simulink model "InvertedPendulum_RealSystem_final"  (R2018a)
settings: Solver=FixedStepDiscrete  StartTime=0.0  StopTime=inf  FixedStep=0.005  RelTol=1e-3
values from neighbouring files (symbols this model uses):
  K_realsetup = lqr(system_open,Q_realsetup,R_realsetup)    [InvertedPendulum.m]
  Omega_c = 25*2*pi    (= 157.079632679)    [InvertedPendulum.m]
  reference_State = [1;0;0;0]    [INVERTEDPENDULUM.m]    (also in InvertedPendulum.m = [0;0;0;0])
  T_s = 1/200    (= 0.005)    [InvertedPendulum.m]
  V_max = 5    [InvertedPendulum.m]
undefined symbols (not defined in the file or in its folder): National_Instruments, PCI
libraries: sldrtlib x2, simulink_extras x1
settings Model: SimulationMode=external  ExtModeTrigDuration=200000  Creator=magudelo  LastModifiedBy=DeKon
settings SolverCC: InsertRTBMode=Always
settings DataIOCC: LimitDataPoints=on  SaveFormat=Array
settings OptimizationCC: ExpressionDepthLimit=2147483647
settings DebuggingCC: UnderspecifiedInitializationDetection=Classic  MergeDetectMultiDrivingBlocksExec=none  SolverPrmCheckMsg=warning  FcnCallInpInsideContextMsg=warning  StateNameClashWarn=warning  SFUnexpectedBacktrackingDiag=warning  SFNoUnconditionalDefaultTransitionDiag=warning  SFExecutionAtInitializationDiag=none
settings ModelReferenceCC: PropagateSignalLabelsOutOfModel=off
settings RTWCC: SystemTargetFile=sldrt.tlc  TemplateMakefile=sldrt.tmf  Description=Simulink Desktop Real-Time  RTWCompilerOptimization=on
settings CodeAppCC: MaxIdLength=95  StateflowObjectComments=on
settings TargetCC: TargetPreCompLibLocation=C:\Program Files\MATLAB\R2018a\toolbox\sldrt\lib\win64  GeneratePreprocessorConditionals=Use local settings
settings ConfigComp: CovMetricSettings=dw  CovHtmlReporting=on  CovSaveCumulativeToWorkspaceVar=on  CovSaveSingleToWorkspaceVar=on  CovExternalEMLEnable=off

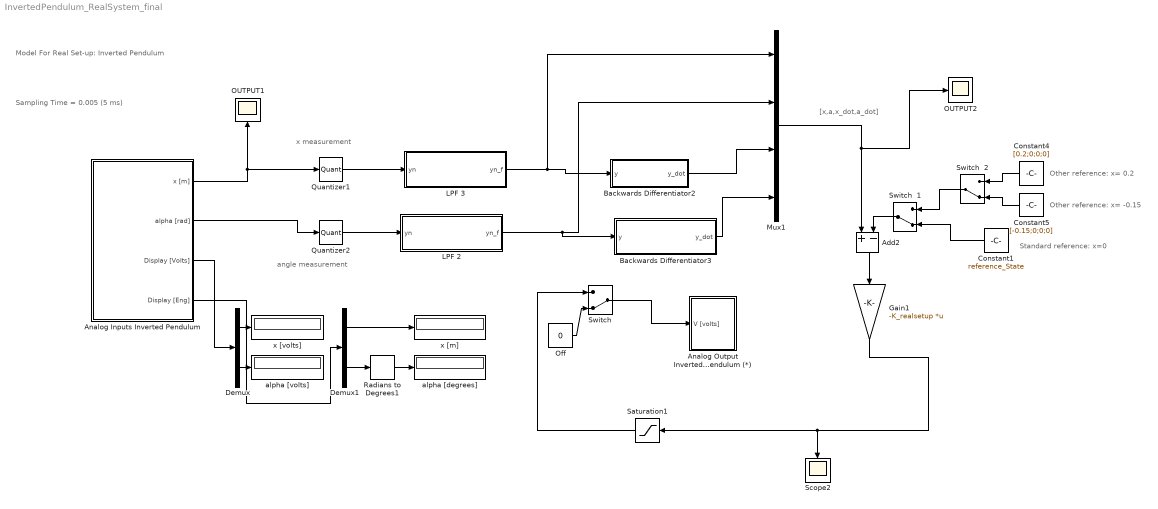
== system InvertedPendulum_RealSystem_final ==
  note: Standard reference: x=0
  note: Other reference: x= 0.2
  note: Model For Real Set-up: Inverted Pendulum
  note: Sampling Time = 0.005 (5 ms)
  note: angle measurement
  note: x measurement
  note: [x,a,x_dot,a_dot]
  note: Other reference: x= -0.15
  Add2 : Sum  Inputs=+-
  Analog Inputs Inverted Pendulum : Subsystem  mask(Analog Inputs. Inverted Pendulum){v2m=0.1033, offset_x=-0.3421, v2r=0.2482, offset_alfa=0.1437}
      mask prompts: v2m "F_x = Convertion factor from Volts to Meters:"; offset_x "Off_x = Offset for the Cart Position [Volts] :"; v2r "F_alpha = Convertion Factor from Volts to Radians :"; offset_alfa "Off_alpha = Offset for the angle of the rob [Volts] :"
      mask help:
      | Remember:
      |    Cart Position (x)           => channel ACH0
      |    Angle of the rod (alpha) => channel ACH1
      |
      |   Cart Position [m] = F_x * ( Cart Position [v] + off_x )
      |   Angle of the rod [rad] = F_alpha * ( Angle of the rod [v] + off_alpha )
  Analog Output Inverted Pendulum (*) : Subsystem  mask(Analog Output - Inverted Pendulum){}
      mask help:
      | Remember
      |    AO 0 => Power Amplifier + Motor
  Backwards Differentiator2 : Subsystem
  Backwards Differentiator3 : Subsystem
  Constant1 : Constant  Value=reference_State
  Constant4 : Constant  Value=[0.2;0;0;0]
  Constant5 : Constant  Value=[-0.15;0;0;0]
  Demux : Demux  Outputs=2
  Demux1 : Demux  Outputs=2
  Gain1 : Gain  Gain=-K_realsetup  Multiplication=Matrix(K*u) (u vector)
  LPF 2 : Subsystem
  LPF 3 : Subsystem
  Mux1 : Mux
  OUTPUT1 : Scope
  OUTPUT2 : Scope
  Off : Constant  Value=0
  Quantizer1 : Quantizer  QuantizationInterval=Q_interval
  Quantizer2 : Quantizer  QuantizationInterval=Q_interval
  Radians to Degrees1 : simulink_extras/Transformations/Radians to Degrees
  Saturation1 : Saturate  UpperLimit=V_max  LowerLimit=-V_max
  Scope2 : Scope
  "Switch  " : ManualSwitch  CurrentSetting=0
  Switch  1 : ManualSwitch  CurrentSetting=0
  Switch  2 : ManualSwitch  CurrentSetting=0
  alpha [degrees] : Display
  alpha [volts] : Display
  x [m] : Display
  x [volts] : Display
  wires:
  Off/1 -> "Switch  "/2
  "Switch  "/1 -> Analog Output Inverted Pendulum (*)/1(V [volts])
  Demux/1 -> x [volts]/1
  Demux1/1 -> x [m]/1
  Demux1/2 -> Radians to Degrees1/1
  Radians to Degrees1/1 -> alpha [degrees]/1
  Analog Inputs Inverted Pendulum/4(Display [Eng]) -> Demux1/1
  Demux/2 -> alpha [volts]/1
  Analog Inputs Inverted Pendulum/3(Display [Volts]) -> Demux/1
  LPF 2/1(yn_f) -> Mux1/2, Backwards Differentiator3/1(y)
  LPF 3/1(yn_f) -> Mux1/1, Backwards Differentiator2/1(y)
  Analog Inputs Inverted Pendulum/2(alpha [rad]) -> Quantizer2/1
  Backwards Differentiator2/1(y_dot) -> Mux1/3
  Analog Inputs Inverted Pendulum/1(x [m]) -> Quantizer1/1, OUTPUT1/1
  Backwards Differentiator3/1(y_dot) -> Mux1/4
  Gain1/1 -> Saturation1/1, Scope2/1
  Mux1/1 -> OUTPUT2/1, Add2/1
  Add2/1 -> Gain1/1
  Saturation1/1 -> "Switch  "/1
  Quantizer1/1 -> LPF 3/1(yn)
  Quantizer2/1 -> LPF 2/1(yn)
  Constant1/1 -> Switch  1/2
  Switch  1/1 -> Add2/2
  Switch  2/1 -> Switch  1/1
  Constant4/1 -> Switch  2/1
  Constant5/1 -> Switch  2/2

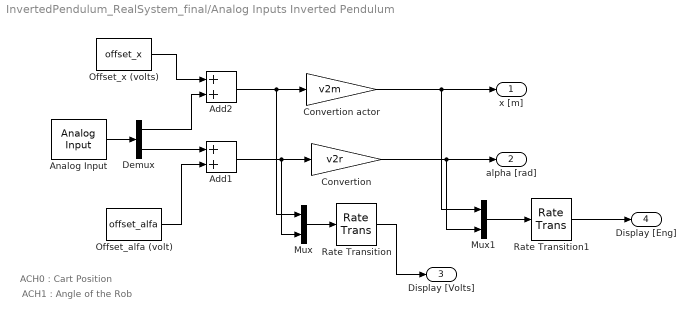
== system InvertedPendulum_RealSystem_final/Analog Inputs Inverted Pendulum ==
  note: ACH0 : Cart Position
  note: ACH1 : Angle of the Rob
  Add1 : Sum
  Add2 : Sum
  Analog Input : sldrtlib/Analog Input  SampleTime=0.005  MaxMissedTicks=10  ShowMissedTicks=off  YieldWhenWaiting=off  DrvName=National_Instruments/PCI-6014  DrvAddress=4294967295  DrvOptions=[1 0 0 0 0 0]  Channels=[1 2]  RangeMode=1  VoltRange=1  DataType=1
      settings: AttributesFormatString=National Instruments\nPCI-6014 [auto]  SourceProductName=Simulink Desktop Real-Time
  "Convertion " : Gain  Gain=v2r
  Convertion actor : Gain  Gain=v2m
  Demux : Demux  Outputs=2
  Mux : Mux  Inputs=2
  Mux1 : Mux  Inputs=2
  Offset_alfa (volt) : Constant  Value=offset_alfa
  Offset_x (volts) : Constant  Value=offset_x
  Rate Transition : RateTransition  OutPortSampleTime=0.25
  Rate Transition1 : RateTransition  OutPortSampleTime=0.25
  x [m] : Outport
  alpha [rad] : Outport  Port=2
  Display [Volts] : Outport  Port=3
  Display [Eng] : Outport  Port=4
  wires:
  Analog Input/1 -> Demux/1
  Demux/1 -> Add2/2
  Add2/1 -> Convertion actor/1, Mux/1
  Offset_x (volts)/1 -> Add2/1
  Convertion actor/1 -> x [m]/1, Mux1/1
  Demux/2 -> Add1/1
  Offset_alfa (volt)/1 -> Add1/2
  Add1/1 -> "Convertion "/1, Mux/2
  "Convertion "/1 -> alpha [rad]/1, Mux1/2
  Mux/1 -> Rate Transition/1
  Rate Transition/1 -> Display [Volts]/1
  Mux1/1 -> Rate Transition1/1
  Rate Transition1/1 -> Display [Eng]/1

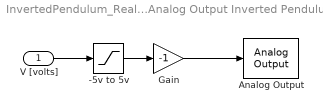
== system InvertedPendulum_RealSystem_final/Analog Output Inverted Pendulum (*) ==
  V [volts] : Inport
  -5v to 5v : Saturate  UpperLimit=5  LowerLimit=-5
  Analog Output : sldrtlib/Analog Output  SampleTime=0.005  MaxMissedTicks=10  ShowMissedTicks=off  YieldWhenWaiting=off  DrvName=National_Instruments/PCI-6014  DrvAddress=4294967295  DrvOptions=[1 0 0 0 0 0]  Channels=1  RangeMode=1  VoltRange=1  InitialValue=0  FinalValue=0
      settings: AttributesFormatString=National Instruments\nPCI-6014 [auto]  SourceProductName=Simulink Desktop Real-Time
  Gain : Gain  Gain=-1
  wires:
  -5v to 5v/1 -> Gain/1
  V [volts]/1 -> -5v to 5v/1
  Gain/1 -> Analog Output/1

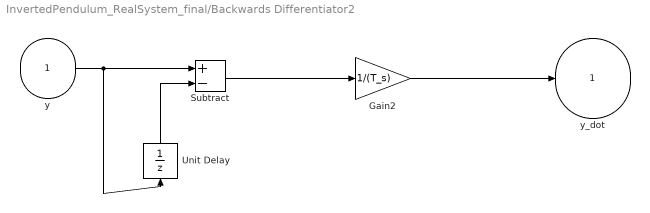
== system InvertedPendulum_RealSystem_final/Backwards Differentiator2 ==
  y : Inport
  Gain2 : Gain  Gain=1/(T_s)
  Subtract : Sum  Inputs=+-
  Unit Delay : UnitDelay  SampleTime=T_s
  y_dot : Outport
  wires:
  y/1 -> Unit Delay/1, Subtract/1
  Unit Delay/1 -> Subtract/2
  Subtract/1 -> Gain2/1
  Gain2/1 -> y_dot/1

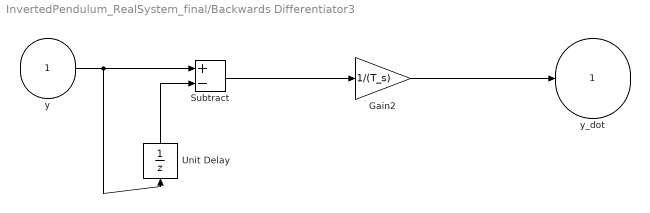
== system InvertedPendulum_RealSystem_final/Backwards Differentiator3 ==
  y : Inport
  Gain2 : Gain  Gain=1/(T_s)
  Subtract : Sum  Inputs=+-
  Unit Delay : UnitDelay  SampleTime=T_s
  y_dot : Outport
  wires:
  Gain2/1 -> y_dot/1
  Subtract/1 -> Gain2/1
  Unit Delay/1 -> Subtract/2
  y/1 -> Subtract/1, Unit Delay/1

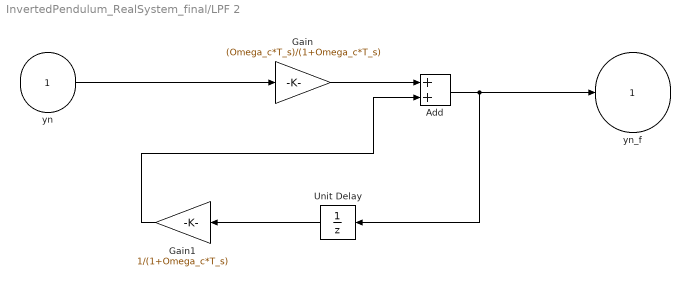
== system InvertedPendulum_RealSystem_final/LPF 2 ==
  yn : Inport
  Add : Sum
  Gain : Gain  Gain=(Omega_c*T_s)/(1+Omega_c*T_s)
  Gain1 : Gain  Gain=1/(1+Omega_c*T_s)
  Unit Delay : UnitDelay  SampleTime=T_s
  yn_f : Outport
  wires:
  Gain1/1 -> Add/2
  Add/1 -> Unit Delay/1, yn_f/1
  Gain/1 -> Add/1
  Unit Delay/1 -> Gain1/1
  yn/1 -> Gain/1

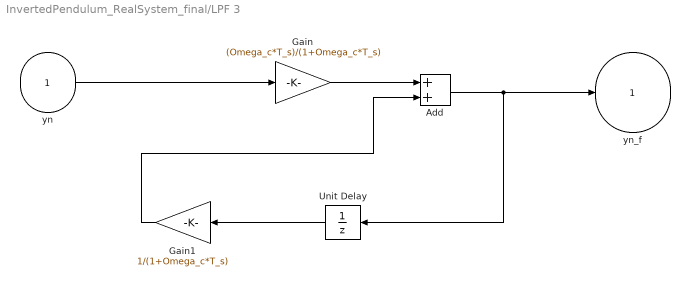
== system InvertedPendulum_RealSystem_final/LPF 3 ==
  yn : Inport
  Add : Sum
  Gain : Gain  Gain=(Omega_c*T_s)/(1+Omega_c*T_s)
  Gain1 : Gain  Gain=1/(1+Omega_c*T_s)
  Unit Delay : UnitDelay  SampleTime=T_s
  yn_f : Outport
  wires:
  yn/1 -> Gain/1
  Unit Delay/1 -> Gain1/1
  Gain/1 -> Add/1
  Add/1 -> Unit Delay/1, yn_f/1
  Gain1/1 -> Add/2
